simulink model "model"  (R2021b)
settings: Solver=VariableStepAuto  StartTime=0.0  StopTime=10.0  RelTol=1e-3
libraries: simulink x1
settings Model: SimulationMode=accelerator  Creator=O  LastModifiedBy=wangzixuan

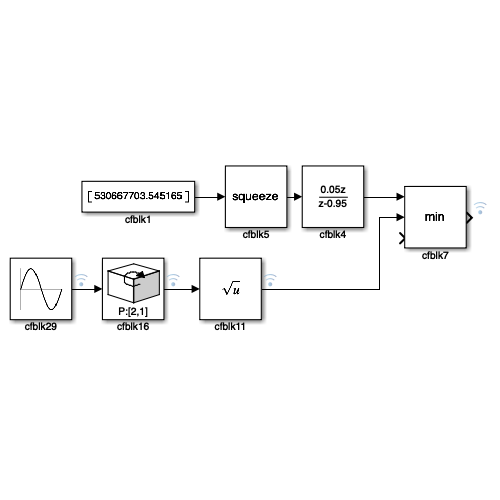
[thumbnail: Simulink's stored preview of the top-level diagram]
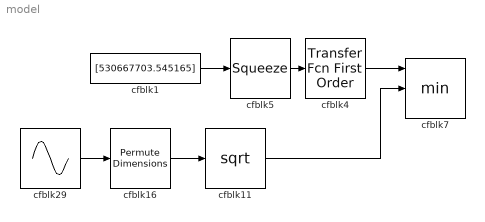
== system model ==
  cfblk1 : Constant  Value=[530667703.545165]  OutDataTypeStr=double  SampleTime=1
  cfblk11 : Sqrt  OutDataTypeStr=double  SaturateOnIntegerOverflow=on
  cfblk16 : PermuteDimensions
  cfblk29 : Sin  Amplitude=[904273925.061287]  Bias=[-144457817.343711]  SampleTime=0
  cfblk4 : simulink/Discrete/Transfer Fcn First Order  PoleZ=0.95  ICPrevOutput=0.0  DoSatur=off
  cfblk5 : Squeeze
  cfblk7 : MinMax  Inputs=3  OutDataTypeStr=double
  wires:
  cfblk11/1 -> cfblk7/2
  cfblk4/1 -> cfblk7/1
  cfblk5/1 -> cfblk4/1
  cfblk16/1 -> cfblk11/1
  cfblk29/1 -> cfblk16/1
  cfblk1/1 -> cfblk5/1
